simulink model "GalvoModel_v3"  (R2013a)
settings: Solver=ode45  StartTime=0.0  StopTime=10.0  RelTol=1e-3
values from neighbouring files (symbols this model uses):
  BEM = 108e-6    (= 0.000108)    [GalvoModel_WOK_step.m]
  CL = 180e-6    (= 0.00018)    [GalvoModel_WOK_step.m]    (also in GalvoModel_v4_sys.m = @(x,n) repmat(x, 1, n); GalvoModel_v6_sys.m = @(x,n) repmat(x, 1, n))
  CR = 2.79    [GalvoModel_WOK_step.m]
  FR = 4e-12    [GalvoModel_WOK_step.m]
  KTR = 47e-3    (= 0.047)    [GalvoModel_WOK_step.m]
  RIN = 1.25e-8    (= 1.25e-08)    [GalvoModel_WOK_step.m]
  TRC = 6.17e-3    (= 0.00617)    [GalvoModel_WOK_step.m]
settings Model: Creator=mainster  LastModifiedBy=mainster
settings DebuggingCC: SolverPrmCheckMsg=none

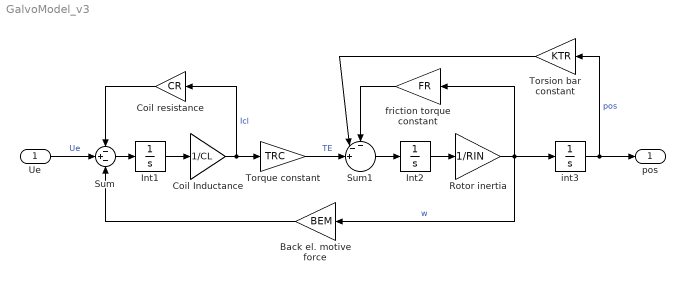
== system GalvoModel_v3 ==
  Ue : Inport
  Back el. motive force : Gain  Gain=BEM
  Coil Inductance : Gain  Gain=1/CL
  Coil resistance : Gain  Gain=CR
  Int1 : Integrator
  Int2 : Integrator
  Rotor inertia : Gain  Gain=1/RIN
  Sum : Sum  Inputs=-+-
  Sum1 : Sum  Inputs=--+||
  Torque constant : Gain  Gain=TRC
  Torsion bar constant : Gain  Gain=KTR
  friction torque constant : Gain  Gain=FR
  int3 : Integrator
  pos : Outport
  wires:
  Sum/1 -> Int1/1
  Rotor inertia/1 -> Back el. motive force/1, int3/1, friction torque constant/1  "w"
  int3/1 -> Torsion bar constant/1, pos/1  "pos"
  Int1/1 -> Coil Inductance/1
  Coil Inductance/1 -> Coil resistance/1, Torque constant/1  "Icl"
  Coil resistance/1 -> Sum/1
  Back el. motive force/1 -> Sum/3
  Int2/1 -> Rotor inertia/1
  friction torque constant/1 -> Sum1/1
  Torsion bar constant/1 -> Sum1/2
  Torque constant/1 -> Sum1/3  "TE"
  Sum1/1 -> Int2/1
  Ue/1 -> Sum/2  "Ue"
